simulink model "mdl_filter_madgwick_16b"  (R2016b)
settings: Solver=ode4  StartTime=0.0  StopTime=10.0  FixedStep=par_filterMadgwick.T  RelTol=1e-3
undefined symbols (not defined in the file or in its folder): Ag_phi_rad, Ag_psi_rad, Ag_theta_rad, AgVel_p_radPerScnd, AgVel_q_radPerScnd, DiscIntNeverNeededParam, fdesignblkfcn, gcbh, Pos_z_mtr, V_w_mtrPerScnd
libraries: dsparch4 x2, dspmathops x1
settings Model: Creator=Nu  LastModifiedBy=Nu

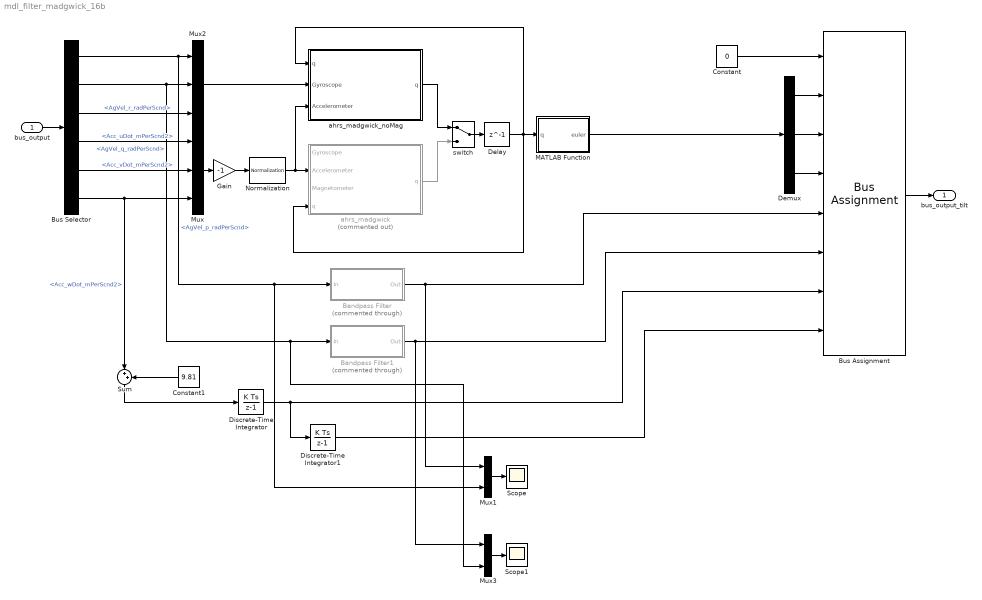
== system mdl_filter_madgwick_16b ==
  bus_output : Inport  OutDataTypeStr=Bus: mdl_output
  Bandpass Filter : Subsystem  Commented=through  DialogController=fdesignblkfcn  InitFcn=fdesignblkfcn(gcbh, {'InitFcn'});  mask(Bandpass Filter){}
      mask help: Design a bandpass filter
      settings: CopyFcn=fdesignblkfcn(gcbh, {'CopyFcn'});
      mask Help: helpview(mapfilelocation('dsp'), 'dspbandpassfilter');
      mask Display: disp('Bandpass');
  Bandpass Filter1 : Subsystem  Commented=through  DialogController=fdesignblkfcn  InitFcn=fdesignblkfcn(gcbh, {'InitFcn'});  mask(Bandpass Filter){}
      mask help: Design a bandpass filter
      settings: CopyFcn=fdesignblkfcn(gcbh, {'CopyFcn'});
      mask Help: helpview(mapfilelocation('dsp'), 'dspbandpassfilter');
      mask Display: disp('Bandpass');
  Bus Assignment : BusAssignment  AssignedSignals=Ag_phi_rad,Ag_theta_rad,Ag_psi_rad,AgVel_p_radPerScnd,AgVel_q_radPerScnd,V_w_mtrPerScnd,Pos_z_mtr
  Bus Selector : BusSelector  OutputSignals=AgVel_p_radPerScnd,AgVel_q_radPerScnd,AgVel_r_radPerScnd,Acc_uDot_mPerScnd2,Acc_vDot_mPerScnd2,Acc_wDot_mPerScnd2
  Constant : Constant  Value=0  OutDataTypeStr=Bus: mdl_statesExt
  Constant1 : Constant  Value=9.81
  Delay : Delay  DelayLength=1  InitialCondition=[1 0 0 0]
  Demux : Demux  Outputs=3
  Discrete-Time Integrator : DiscreteIntegrator  InitialConditionSetting=State (most efficient)  SampleTime=-1  ICPrevOutput=DiscIntNeverNeededParam  ICPrevScaledInput=DiscIntNeverNeededParam
  Discrete-Time Integrator1 : DiscreteIntegrator  InitialConditionSetting=State (most efficient)  SampleTime=-1  ICPrevOutput=DiscIntNeverNeededParam  ICPrevScaledInput=DiscIntNeverNeededParam
  Gain : Gain  Gain=-1
  MATLAB Function : MATLAB Function  TreatAsAtomicUnit=on
  Mux : Mux  Inputs=3
  Mux1 : Mux  Inputs=2
  Mux2 : Mux  Inputs=3
  Mux3 : Mux  Inputs=2
  Normalization : dspmathops/Normalization  NormType=Squared 2-norm  Bias=1e-10  NormOver=Each column  Dimension=1  outputDataTypeStr=Inherit: Same as product output  outputLastDataTypeStr=Inherit: Same as product output  outputMin=[]  outputMax=[]  accumDataTypeStr=Inherit: Same as product output  accumLastDataTypeStr=Inherit: Same as product output  roundingMode=Floor  overflowMode=off
  Scope : Scope
  Scope1 : Scope
  Sum : Sum  Inputs=|++
  ahrs_madgwick : MATLAB Function  Commented=on  TreatAsAtomicUnit=on
  ahrs_madgwick_noMag : MATLAB Function  TreatAsAtomicUnit=on
  switch : ManualSwitch
  "bus_output_tilt " : Outport  OutDataTypeStr=Bus: mdl_statesExt
  wires:
  bus_output/1 -> Bus Selector/1
  Bus Selector/4 -> Mux/1  "<Acc_uDot_mPerScnd2>"
  Bus Selector/5 -> Mux/2  "<Acc_vDot_mPerScnd2>"
  Bus Selector/6 -> Sum/1, Mux/3  "<Acc_wDot_mPerScnd2>"
  Bus Selector/3 -> Mux2/3  "<AgVel_r_radPerScnd>"
  Constant/1 -> Bus Assignment/1
  Bus Assignment/1 -> "bus_output_tilt "/1
  Mux/1 -> Gain/1
  switch/1 -> Delay/1
  ahrs_madgwick/1(q) -> switch/2
  ahrs_madgwick_noMag/1(q) -> switch/1
  Delay/1 -> ahrs_madgwick/4("q "), MATLAB Function/1(q), ahrs_madgwick_noMag/1("q ")
  Normalization/1 -> ahrs_madgwick/2(Accelerometer), ahrs_madgwick_noMag/3(Accelerometer)
  MATLAB Function/1(euler) -> Demux/1
  Demux/1 -> Bus Assignment/2
  Demux/2 -> Bus Assignment/3
  Demux/3 -> Bus Assignment/4
  Mux2/1 -> ahrs_madgwick_noMag/2(Gyroscope)
  Gain/1 -> Normalization/1
  Bus Selector/1 -> Mux2/1, Mux1/2, Bandpass Filter/1(In)  "<AgVel_p_radPerScnd>"
  Discrete-Time Integrator/1 -> Discrete-Time Integrator1/1, Bus Assignment/7
  Discrete-Time Integrator1/1 -> Bus Assignment/8
  Sum/1 -> Discrete-Time Integrator/1
  Constant1/1 -> Sum/2
  Bandpass Filter/1(Out) -> Mux1/1, Bus Assignment/5
  Mux1/1 -> Scope/1
  Bus Selector/2 -> Mux2/2, Bandpass Filter1/1(In), Mux3/2  "<AgVel_q_radPerScnd>"
  Bandpass Filter1/1(Out) -> Mux3/1, Bus Assignment/6
  Mux3/1 -> Scope1/1

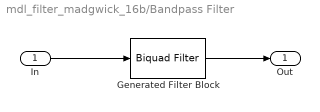
== system mdl_filter_madgwick_16b/Bandpass Filter ==
  In : Inport
  Generated Filter Block : dsparch4/Biquad Filter  Tag=BlockMethodSubSystem  IIRFiltStruct=Direct form II  CoeffSource=Specify via dialog  BiQuadCoeffs=[0.094070781761715877 0 -0.094070781761715877 1 -0.6042278333076686 0.31945550818977708;1.084867434642782 0 -1.084867434642782 1 -1.4063774988099191 0.81935005133372041;0.24695674108127819 0 -0.24695674108127819 1 0.06632880507369382 0.72950157169404795;0.70689638081876904 0 -0.70689638081876904 1 -1.0643670918246446 0.52235369338964377;0.70593237126682085 0 -0.70593237126682085 1 -0.17152930636953417 0.39324226162320108]  a0Flag=Warning  IC=0  ICnum=0  ICden=0  InputProcessing=Columns as channels (frame based)  denAccumFracLength=30  denProdOutputFracLength=30  secondMemoryFracLength=15  roundingMode=Floor  overflowMode=off  ScaleValues=[0.57516530669323129;1;1;1;1;1]  optimizeScaleValues=off  ScaleValueMode=Specify via input port (g)  scaleValueFracLength=14  FilterSource=Specify via dialog  FilterObject=BQF
  Out : Outport
  wires:
  In/1 -> Generated Filter Block/1
  Generated Filter Block/1 -> Out/1

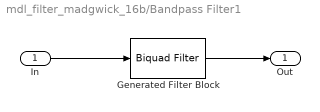
== system mdl_filter_madgwick_16b/Bandpass Filter1 ==
  In : Inport
  Generated Filter Block : dsparch4/Biquad Filter  Tag=BlockMethodSubSystem  IIRFiltStruct=Direct form II  CoeffSource=Specify via dialog  BiQuadCoeffs=[0.094070781761715877 0 -0.094070781761715877 1 -0.6042278333076686 0.31945550818977708;1.084867434642782 0 -1.084867434642782 1 -1.4063774988099191 0.81935005133372041;0.24695674108127819 0 -0.24695674108127819 1 0.06632880507369382 0.72950157169404795;0.70689638081876904 0 -0.70689638081876904 1 -1.0643670918246446 0.52235369338964377;0.70593237126682085 0 -0.70593237126682085 1 -0.17152930636953417 0.39324226162320108]  a0Flag=Warning  IC=0  ICnum=0  ICden=0  InputProcessing=Columns as channels (frame based)  denAccumFracLength=30  denProdOutputFracLength=30  secondMemoryFracLength=15  roundingMode=Floor  overflowMode=off  ScaleValues=[0.57516530669323129;1;1;1;1;1]  optimizeScaleValues=off  ScaleValueMode=Specify via input port (g)  scaleValueFracLength=14  FilterSource=Specify via dialog  FilterObject=BQF
  Out : Outport
  wires:
  Generated Filter Block/1 -> Out/1
  In/1 -> Generated Filter Block/1

== matlab function mdl_filter_madgwick_16b/ahrs_madgwick_noMag ==
  data: q input; Gyroscope input; q output; Accelerometer input; par_filterMadgwick parameter
function q = fcn(q, Gyroscope, Accelerometer, par_filterMadgwick)

% Gradient decent algorithm corrective step
F = [2*(q(2)*q(4) - q(1)*q(3)) - Accelerometer(1)
    2*(q(1)*q(2) + q(3)*q(4)) - Accelerometer(2)
    2*(0.5 - q(2)^2 - q(3)^2) - Accelerometer(3)];
J = [-2*q(3),	2*q(4),    -2*q(1),	2*q(2)
    2*q(2),     2*q(1),     2*q(4),	2*q(3)
    0,         -4*q(2),    -4*q(3),	0    ];
step = (J'*F);
step = step / norm(step);	% normalise step magnitude

% Compute rate of change of quaternion
qDot = 0.5 * quaternProd(q.', [0 Gyroscope(1) Gyroscope(2) Gyroscope(3)]) - par_filterMadgwick.beta * step';
qDot = qDot.';

% Integrate to yield quaternion
q = q + qDot * par_filterMadgwick.T;
q = q / norm(q); % normalise quaternion

== matlab function mdl_filter_madgwick_16b/ahrs_madgwick ==
  data: Gyroscope input; Accelerometer input; Magnetometer input; q input; q output; par_filterMadgwick parameter
function q = fcn(Gyroscope, Accelerometer, Magnetometer, q, par_filterMadgwick)

% Reference direction of Earth's magnetic feild
h = quaternProd(q, quaternProd([0 Magnetometer], quaternConj(q)));
b = [0 norm([h(2) h(3)]) 0 h(4)];

% Gradient decent algorithm corrective step
F = [2*(q(2)*q(4) - q(1)*q(3)) - Accelerometer(1)
    2*(q(1)*q(2) + q(3)*q(4)) - Accelerometer(2)
    2*(0.5 - q(2)^2 - q(3)^2) - Accelerometer(3)
    2*b(2)*(0.5 - q(3)^2 - q(4)^2) + 2*b(4)*(q(2)*q(4) - q(1)*q(3)) - Magnetometer(1)
    2*b(2)*(q(2)*q(3) - q(1)*q(4)) + 2*b(4)*(q(1)*q(2) + q(3)*q(4)) - Magnetometer(2)
    2*b(2)*(q(1)*q(3) + q(2)*q(4)) + 2*b(4)*(0.5 - q(2)^2 - q(3)^2) - Magnetometer(3)];
J = [-2*q(3),                 	2*q(4),                    -2*q(1),                         2*q(2)
    2*q(2),                 	2*q(1),                    	2*q(4),                         2*q(3)
    0,                         -4*q(2),                    -4*q(3),                         0
    -2*b(4)*q(3),               2*b(4)*q(4),               -4*b(2)*q(3)-2*b(4)*q(1),       -4*b(2)*q(4)+2*b(4)*q(2)
    -2*b(2)*q(4)+2*b(4)*q(2),	2*b(2)*q(3)+2*b(4)*q(1),	2*b(2)*q(2)+2*b(4)*q(4),       -2*b(2)*q(1)+2*b(4)*q(3)
    2*b(2)*q(3),                2*b(2)*q(4)-4*b(4)*q(2),	2*b(2)*q(1)-4*b(4)*q(3),        2*b(2)*q(2)];
step = (J'*F);
step = step / norm(step);	% normalise step magnitude

% Compute rate of change of quaternion
qDot = 0.5 * quaternProd(q, [0 Gyroscope(1) Gyroscope(2) Gyroscope(3)]) - par_filterMadgwick.beta * step';

% Integrate to yield quaternion
q = q + qDot * par_filterMadgwick.T;
q = q / norm(q); % normalise quaternion

== matlab function mdl_filter_madgwick_16b/MATLAB Function ==
  data: q input; euler output
function euler = fcn(q)

euler = quatern2euler(quaternConj(q.'));
